simulink model "blaanisser_vs_rodnisser"  (R2018a)
settings: Solver=VariableStepAuto  StartTime=0.0  StopTime=60  RelTol=1e-3
libraries: simulink x6, dspsrcs4 x1
settings Model: Creator=gustavoo  LastModifiedBy=gustavoo
settings SolverCC: ZeroCrossControl=DisableAll

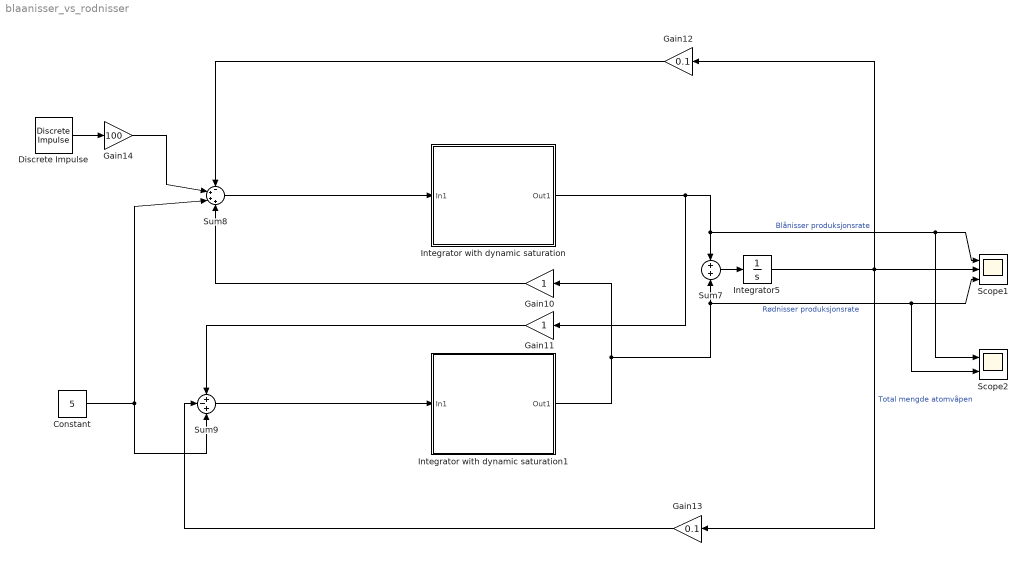
== system blaanisser_vs_rodnisser ==
  Constant : Constant  Value=5
  Discrete Impulse : dspsrcs4/Discrete  Impulse  Delay=0  SampleTime=1  FrameSample=1  OutputFrames=off  dataType=double  isSigned=on  wordLen=16  udDataType=sfix(16)  fracBitsMode=Best precision  numFracBits=15  OutDataTypeStr=double  LastOutDataTypeStr=double
  Gain10 : Gain
  Gain11 : Gain
  Gain12 : Gain  Gain=0.1
  Gain13 : Gain  Gain=0.1
  Gain14 : Gain  Gain=100
  Integrator with dynamic saturation : Subsystem
  Integrator with dynamic saturation1 : Subsystem
  Integrator5 : Integrator  LimitOutput=on  LowerSaturationLimit=0
  Scope1 : Scope  NumInputPorts=3
  Scope2 : Scope  NumInputPorts=2
  Sum7 : Sum  Inputs=+|+
  Sum8 : Sum  Inputs=-+++
  Sum9 : Sum  Inputs=+-+
  wires:
  Integrator with dynamic saturation1/1(Out1) -> Scope2/2, Scope1/3, Sum7/2, Gain10/1  "Rødnisser produksjonsrate"
  Integrator with dynamic saturation/1(Out1) -> Scope2/1, Scope1/1, Sum7/1, Gain11/1  "Blånisser produksjonsrate"
  Gain14/1 -> Sum8/2
  Gain12/1 -> Sum8/1
  Sum9/1 -> Integrator with dynamic saturation1/1(In1)
  Discrete Impulse/1 -> Gain14/1
  Integrator5/1 -> Gain13/1, Gain12/1, Scope1/2  "Total mengde atomvåpen"
  Gain11/1 -> Sum9/1
  Gain13/1 -> Sum9/2
  Gain10/1 -> Sum8/4
  Constant/1 -> Sum8/3, Sum9/3
  Sum8/1 -> Integrator with dynamic saturation/1(In1)
  Sum7/1 -> Integrator5/1

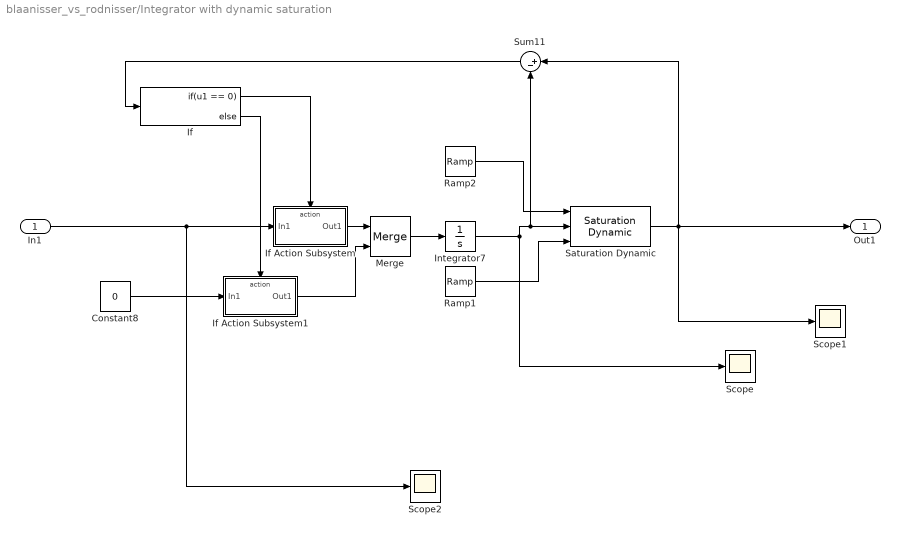
== system blaanisser_vs_rodnisser/Integrator with dynamic saturation ==
  In1 : Inport
  Constant8 : Constant  Value=0
  If : If  IfExpression=u1 == 0
  If Action Subsystem : Subsystem  TreatAsAtomicUnit=on
  If Action Subsystem1 : Subsystem  TreatAsAtomicUnit=on
  Integrator7 : Integrator  ZeroCross=off
  Merge : Merge
  Ramp1 : simulink/Sources/Ramp  slope=-0.1  start=0  InitialOutput=0
  Ramp2 : simulink/Sources/Ramp  slope=1  start=0  InitialOutput=0
  Saturation Dynamic : simulink/Discontinuities/Saturation Dynamic  OutMin=[]  OutMax=[]  OutDataTypeStr=Inherit: Same as second input  OutDataType=fixdt(1, 16)  OutScaling=2^-10  DoSatur=off
  Scope : Scope
  Scope1 : Scope
  Scope2 : Scope
  Sum11 : Sum  Inputs=|+-
  Out1 : Outport
  wires:
  Constant8/1 -> If Action Subsystem1/1(In1)
  Integrator7/1 -> Saturation Dynamic/2, Sum11/2, Scope/1
  Saturation Dynamic/1 -> Scope1/1, Out1/1, Sum11/1
  Ramp1/1 -> Saturation Dynamic/3
  Ramp2/1 -> Saturation Dynamic/1
  Sum11/1 -> If/1
  If/2 -> If Action Subsystem1/Action
  In1/1 -> Scope2/1, If Action Subsystem/1(In1)
  If/1 -> If Action Subsystem/Action
  Merge/1 -> Integrator7/1
  If Action Subsystem/1(Out1) -> Merge/1
  If Action Subsystem1/1(Out1) -> Merge/2

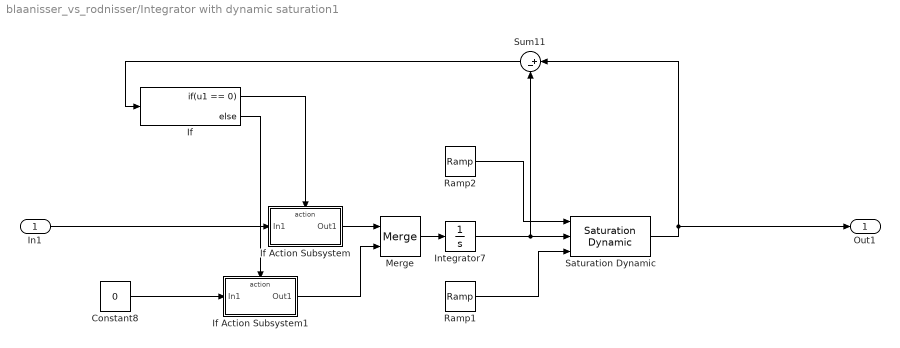
== system blaanisser_vs_rodnisser/Integrator with dynamic saturation1 ==
  In1 : Inport
  Constant8 : Constant  Value=0
  If : If  IfExpression=u1 == 0
  If Action Subsystem : Subsystem  TreatAsAtomicUnit=on
  If Action Subsystem1 : Subsystem  TreatAsAtomicUnit=on
  Integrator7 : Integrator  ZeroCross=off
  Merge : Merge
  Ramp1 : simulink/Sources/Ramp  slope=-0.1  start=0  InitialOutput=0
  Ramp2 : simulink/Sources/Ramp  slope=1  start=0  InitialOutput=0
  Saturation Dynamic : simulink/Discontinuities/Saturation Dynamic  OutMin=[]  OutMax=[]  OutDataTypeStr=Inherit: Same as second input  OutDataType=fixdt(1, 16)  OutScaling=2^-10  DoSatur=off
  Sum11 : Sum  Inputs=|+-
  Out1 : Outport
  wires:
  Constant8/1 -> If Action Subsystem1/1(In1)
  Integrator7/1 -> Sum11/2, Saturation Dynamic/2
  Saturation Dynamic/1 -> Out1/1, Sum11/1
  Ramp1/1 -> Saturation Dynamic/3
  Ramp2/1 -> Saturation Dynamic/1
  Sum11/1 -> If/1
  If/2 -> If Action Subsystem1/Action
  In1/1 -> If Action Subsystem/1(In1)
  If/1 -> If Action Subsystem/Action
  If Action Subsystem/1(Out1) -> Merge/1
  If Action Subsystem1/1(Out1) -> Merge/2
  Merge/1 -> Integrator7/1

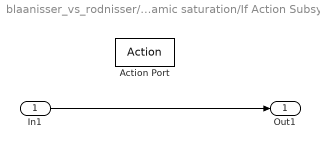
== system blaanisser_vs_rodnisser/Integrator with dynamic saturation/If Action Subsystem ==
  In1 : Inport
  Action Port : ActionPort  ActionType=then
  Out1 : Outport
  wires:
  In1/1 -> Out1/1

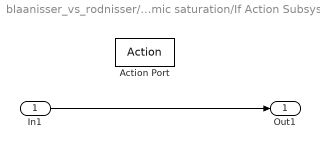
== system blaanisser_vs_rodnisser/Integrator with dynamic saturation/If Action Subsystem1 ==
  In1 : Inport
  Action Port : ActionPort  ActionType=else
  Out1 : Outport
  wires:
  In1/1 -> Out1/1

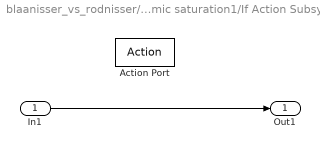
== system blaanisser_vs_rodnisser/Integrator with dynamic saturation1/If Action Subsystem ==
  In1 : Inport
  Action Port : ActionPort  ActionType=then
  Out1 : Outport
  wires:
  In1/1 -> Out1/1

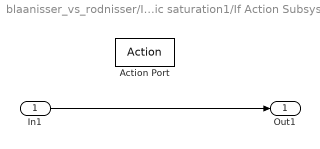
== system blaanisser_vs_rodnisser/Integrator with dynamic saturation1/If Action Subsystem1 ==
  In1 : Inport
  Action Port : ActionPort  ActionType=else
  Out1 : Outport
  wires:
  In1/1 -> Out1/1
